simulink model "final_quadruped_120722"  (R2021a)
settings: Solver=ode15s  StartTime=0.0  StopTime=10  FixedStep=1e-3  RelTol=1e-5  EnableMultiTasking=on
values from neighbouring files (symbols this model uses):
  foot_x = 8    [bipedparameters.m]    (also in fcn.m; finalrobotParameters.m; finalrobotParameters_110522.m; finalrobotParameters_140522.m)
  foot_y = 6    [bipedparameters.m]    (also in fcn.m; finalrobotParameters.m; finalrobotParameters_110522.m; finalrobotParameters_140522.m)
  foot_z = 1    [bipedparameters.m]    (also in fcn.m; finalrobotParameters.m; finalrobotParameters_110522.m; finalrobotParameters_140522.m)
  height_plane = 0.025    [bipedparameters.m]    (also in finalrobotParameters.m; finalrobotParameters_110522.m; finalrobotParameters_140522.m; finalrobotParameters_240522.m)
  kd_ankle = 1000    [bipedparameters.m]    (also in finalrobotParameters_240522.m)
  kd_hip = 1000    [bipedparameters.m]    (also in finalrobotParameters_240522.m)
  kd_knee = 1000    [bipedparameters.m]    (also in finalrobotParameters_240522.m)
  ki_ankle = 1000    [bipedparameters.m]    (also in finalrobotParameters_240522.m)
  ki_hip = 1000    [bipedparameters.m]    (also in finalrobotParameters_240522.m)
  ki_knee = 2000    [bipedparameters.m]    (also in finalrobotParameters_240522.m)
  kp_ankle = 1000    [bipedparameters.m]    (also in finalrobotParameters_240522.m)
  kp_hip = 1000    [bipedparameters.m]    (also in finalrobotParameters_240522.m)
  kp_knee = 2000    [bipedparameters.m]    (also in finalrobotParameters_240522.m)
  lower_leg_length = 10    [bipedparameters.m]    (also in fcn.m; finalrobotParameters.m; finalrobotParameters_110522.m; finalrobotParameters_140522.m)
  plane_x = 25    [bipedparameters.m]    (also in finalrobotParameters.m; finalrobotParameters_110522.m; finalrobotParameters_140522.m; finalrobotParameters_240522.m)
  plane_y = 3    [bipedparameters.m]    (also in finalrobotParameters.m; finalrobotParameters_110522.m; finalrobotParameters_140522.m; finalrobotParameters_240522.m)
  torso_offset_x = -0.5    [bipedparameters.m]    (also in finalrobotParameters.m = 10; finalrobotParameters_110522.m = 10; finalrobotParameters_140522.m = 10; finalrobotParameters_240522.m = 10)
  torso_offset_z = -2    [bipedparameters.m]    (also in finalrobotParameters.m; finalrobotParameters_110522.m; finalrobotParameters_140522.m; finalrobotParameters_240522.m)
  torso_x = 5    [bipedparameters.m]    (also in fcn.m = 25; finalrobotParameters.m = 25; finalrobotParameters_110522.m = 25; finalrobotParameters_140522.m = 25)
  torso_y = 10    [bipedparameters.m]    (also in fcn.m = 16; finalrobotParameters.m = 16; finalrobotParameters_110522.m = 16; finalrobotParameters_140522.m = 16)
  torso_z = 8    [bipedparameters.m]    (also in fcn.m = 10; finalrobotParameters.m = 10; finalrobotParameters_110522.m = 10; finalrobotParameters_140522.m = 10)
  upper_leg_length = 10    [bipedparameters.m]    (also in fcn.m; finalrobotParameters.m; finalrobotParameters_110522.m; finalrobotParameters_140522.m)
undefined symbols (not defined in the file or in its folder): sigbuilder_block, X, Y, Z
libraries: nesl_utility x288, sm_lib x75, pid_lib x20, Contact_Forces_Lib x16, fl_lib x3
(part 4 of 9)

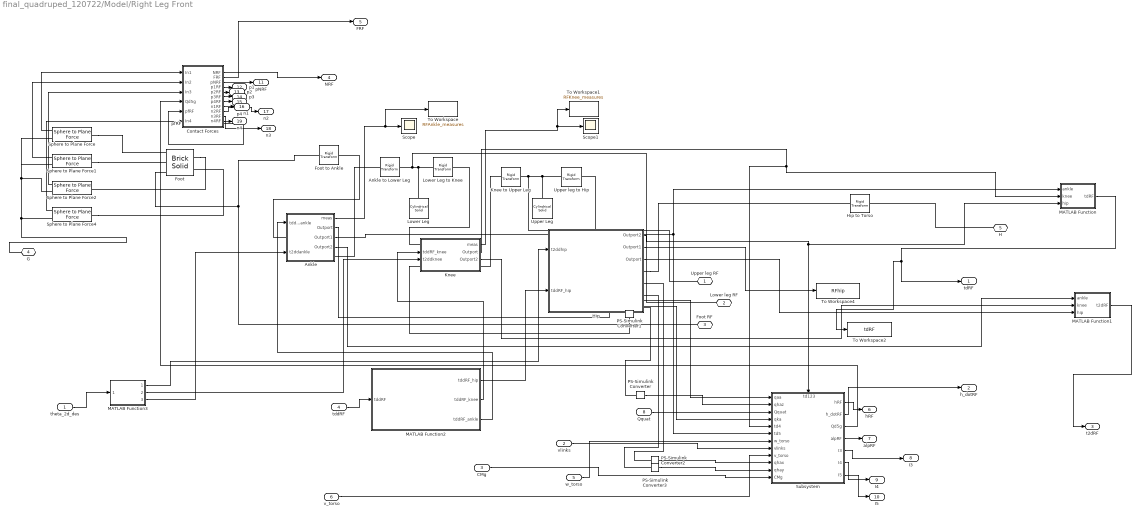
== system final_quadruped_120722/Model/Right Leg Front  ==
  theta_2d_des : Inport
  vlinks : Inport  Port=2
  CMg : Inport  Port=3
  tddRF : Inport  Port=4
  w_torso : Inport  Port=5
  v_torso : Inport  Port=6
  pfRF : Inport  Port=7
  Qquat : Inport  Port=8
  "Ankle " : Subsystem
      settings: PortSchema="{\"entries\":[{\"content\":{\"sides\":[{\"content\":{\"connectorIds\":[\"In1\",\"LConn1\",\"In2\"]},\"type\":\"ConnectorPlacement.EquallySpacedRectSide\",\"uuid\":\"8820d672-3cef-4e81-999d-8ce69d7112c4\"},{\"content\":{\"connectorIds\":[\"Out1\",\"Out2\",\"Out3\",\"Out4\",\"RConn1\"],\"side\":\"RIGHT\"},\"type\":\"ConnectorPlacement.EquallySpacedRectSide\",\"uuid\":\"2ab010ff-dc37-45a7-8249-0a0b10f28039\"},{\"content\":{\"connectorIds\":[],\"side\":\"TOP\"},\"type\":\"ConnectorPlacement.EquallySpacedRectSide\",\"uuid\":\"2949f9ef-a473-4fca-9f6b-f5ba56dbec95\"}]},\"type\":\"ConnectorPlacement.EquallySpacedConnector\",\"uuid\":\"7b6aa300-a222-434d-a157-d54fa47a17c2\"}],\"packageUris\":[\"http://schema.mathworks.com/mf0/Connector/R2020b\"],\"version\":\"1.0\"}"
  Ankle to Lower Leg : sm_lib/Frames and Transforms/Rigid Transform  TranslationMethod=Cartesian  TranslationStandardOffset=5  TranslationLengthUnit=cm  TranslationStandardAxis=+Y  TranslationCartesianOffset=[0 lower_leg_length/2 0]  TranslationROffset=0  TranslationROffsetUnits=m  TranslationZOffset=0  TranslationZOffsetUnits=m  TranslationThetaOffset=0  TranslationThetaOffsetUnits=deg  RotationMethod=StandardAxis  RotationAngleUnits=deg  RotationStandardAxis=-X  RotationAngle=90  RotationArbitraryAxis=[0 0 1]  FollAlignAxisA=+X  BaseAlignAxisA=+Y  FollAlignAxisB=+Y  BaseAlignAxisB=+Z  RotationSequenceAxes=FollowerAxes  RotationSequence=XYX  RotationSequenceAngles=[0 0 0]  RotationSequenceAnglesUnits=deg  RotationMatrix=[1 0 0; 0 1 0; 0 0 1]
  "Contact Forces " : Subsystem
  Foot : sm_lib/Body Elements/Brick Solid  GraphicAmbientColor=[0.15 0.15 0.15 1.0]  BasedOnType=Density  BrickDimensions=[foot_x foot_y foot_z]  BrickDimensionUnits=cm  CenterOfMass=[0 0 0]  CenterOfMassUnits=m  GraphicDiffuseColor=[0.5 0.5 0.5]  Density=foot_density  DensityUnits=kg/m^3  DoExposeReferenceFrame=off  GraphicEmissiveColor=[0.0 0.0 0.0 1.0]  ExportEntireGeometry=off  SerializedFrames=<Frames><Frame><Id>Frame1</Id><Value><Name>F1</Name><Origin><Source>GeometricFeature</Source><FeatureName>+x -y -z point</FeatureName></Origin><PrimaryAxis><DefinedDirection>+Z</DefinedDirection><Source>ReferenceFrame</Source><SourceDirection>+Z</SourceDirection><FeatureName></FeatureName></PrimaryAxis><SecondaryAxis><DefinedDirection>+X</DefinedDirection><Source>ReferenceFrame</Source><SourceDirection>+X</SourceDirection><FeatureName></FeatureName></SecondaryAxis></Value></Frame><Frame><Id>Frame2</Id><Value><Name>F2</Name><Origin><Source>GeometricFeature</Source><FeatureName>-x -y -z point</FeatureName></Origin><PrimaryAxis><DefinedDirection>+Z</DefinedDirection><Source>ReferenceFrame</Source><SourceDirection>+Z</SourceDirection><FeatureName></FeatureName></PrimaryAxis><SecondaryAxis><DefinedDirection>+X</DefinedDirection><Source>ReferenceFrame</Source><SourceDirection>+X</SourceDirection><FeatureName></FeatureName></SecondaryAxis></Value></Frame><Frame><Id>Frame3</Id><Value><Name>F3</Name><Origin><Source>GeometricFeature</Source><FeatureName>+x +y -z point</FeatureName></Origin><PrimaryAxis><DefinedDirection>+Z</DefinedDirection><Source>ReferenceFrame</Source><SourceDirection>+Z</SourceDirection><FeatureName></FeatureName></PrimaryAxis><SecondaryAxis><DefinedDirection>+X</DefinedDirection><Source>ReferenceFrame</Source><SourceDirection>+X</SourceDirection><FeatureName></FeatureName></SecondaryAxis></Value></Frame><Frame><Id>Frame4</Id><Value><Name>F4</Name><Origin><Source>GeometricFeature</Source><FeatureName>-x +y -z point</FeatureName></Origin><PrimaryAxis><DefinedDirection>+Z</DefinedDirection><Source>ReferenceFrame</Source><SourceDirection>+Z</SourceDirection><FeatureName></FeatureName></PrimaryAxis><SecondaryAxis><DefinedDirection>+X</DefinedDirection><Source>ReferenceFrame</Source><SourceDirection>+X</SourceDirection><FeatureName></FeatureName></SecondaryAxis></Value></Frame><Frame><Id>Frame5</Id><Value><Name>B</Name><Origin><Source>GeometricFeature</Source><FeatureName>+z surface</FeatureName></Origin><PrimaryAxis><DefinedDirection>+Z</DefinedDirection><Source>ReferenceFrame</Source><SourceDirection>-Y</SourceDirection><FeatureName></FeatureName></PrimaryAxis><SecondaryAxis><DefinedDirection>+X</DefinedDirection><Source>ReferenceFrame</Source><SourceDirection>+X</SourceDirection><FeatureName></FeatureName></SecondaryAxis></Value></Frame></Frames>  MarkerShape=Sphere  MarkerSize=10  GraphicType=FromGeometry  InertiaType=CalculateFromGeometry  Mass=1  MassUnits=kg  MomentsOfInertia=[1 1 1]  MomentsOfInertiaUnits=kg*m^2  GraphicOpacity=1.0  ProductsOfInertia=[1 1 1]  ProductsOfInertiaUnits=kg*m^2  GraphicShininess=75  GraphicSpecularColor=[0.5 0.5 0.5 1.0]  GraphicVisPropType=SimpleVisualProperties
  Foot to Ankle : sm_lib/Frames and Transforms/Rigid Transform  TranslationMethod=Cartesian  TranslationStandardOffset=0  TranslationLengthUnit=cm  TranslationStandardAxis=+Z  TranslationCartesianOffset=foot_offset  TranslationROffset=0  TranslationROffsetUnits=m  TranslationZOffset=0  TranslationZOffsetUnits=m  TranslationThetaOffset=0  TranslationThetaOffsetUnits=deg  RotationMethod=None  RotationAngleUnits=deg  RotationStandardAxis=+X  RotationAngle=90  RotationArbitraryAxis=[0 0 1]  FollAlignAxisA=+X  BaseAlignAxisA=+Y  FollAlignAxisB=+Y  BaseAlignAxisB=+Z  RotationSequenceAxes=FollowerAxes  RotationSequence=XYX  RotationSequenceAngles=[0 0 0]  RotationSequenceAnglesUnits=deg  RotationMatrix=[1 0 0; 0 1 0; 0 0 1]
  Hip : Subsystem
      settings: PortSchema="{\"entries\":[{\"content\":{\"sides\":[{\"content\":{\"connectorIds\":[\"In1\",\"In2\"]},\"type\":\"ConnectorPlacement.EquallySpacedRectSide\",\"uuid\":\"3c672348-e331-4589-83a8-aa84cb04ec22\"},{\"content\":{\"connectorIds\":[\"Out1\",\"Out2\",\"Out3\",\"RConn1\",\"RConn2\",\"RConn3\",\"RConn4\"],\"side\":\"RIGHT\"},\"type\":\"ConnectorPlacement.EquallySpacedRectSide\",\"uuid\":\"0cc20eac-f861-4ef7-921b-23889a7eea47\"},{\"content\":{\"connectorIds\":[\"LConn1\"],\"side\":\"TOP\"},\"type\":\"ConnectorPlacement.EquallySpacedRectSide\",\"uuid\":\"90940c46-a35e-4cbd-8c5c-08301adb8b47\"}]},\"type\":\"ConnectorPlacement.EquallySpacedConnector\",\"uuid\":\"ac1266b5-f3f5-41bb-99c9-3c0745f7848a\"}],\"packageUris\":[\"http://schema.mathworks.com/mf0/Connector/R2020b\"],\"version\":\"1.0\"}"
  Hip to Torso : sm_lib/Frames and Transforms/Rigid Transform  TranslationMethod=None  TranslationStandardOffset=0  TranslationLengthUnit=m  TranslationStandardAxis=+Z  TranslationCartesianOffset=[0 0 0]  TranslationROffset=0  TranslationROffsetUnits=m  TranslationZOffset=0  TranslationZOffsetUnits=m  TranslationThetaOffset=0  TranslationThetaOffsetUnits=deg  RotationMethod=StandardAxis  RotationAngleUnits=deg  RotationStandardAxis=+X  RotationAngle=-90  RotationArbitraryAxis=[0 0 1]  FollAlignAxisA=+X  BaseAlignAxisA=+Y  FollAlignAxisB=+Y  BaseAlignAxisB=+Z  RotationSequenceAxes=FollowerAxes  RotationSequence=XYX  RotationSequenceAngles=[0 0 0]  RotationSequenceAnglesUnits=deg  RotationMatrix=[1 0 0; 0 1 0; 0 0 1]
  Knee : Subsystem
      settings: PortSchema="{\"entries\":[{\"content\":{\"sides\":[{\"content\":{\"connectorIds\":[\"LConn1\",\"In1\",\"In2\",\"LConn2\"]},\"type\":\"ConnectorPlacement.EquallySpacedRectSide\",\"uuid\":\"3c672348-e331-4589-83a8-aa84cb04ec22\"},{\"content\":{\"connectorIds\":[\"Out1\",\"Out2\",\"Out3\",\"RConn1\"],\"side\":\"RIGHT\"},\"type\":\"ConnectorPlacement.EquallySpacedRectSide\",\"uuid\":\"0cc20eac-f861-4ef7-921b-23889a7eea47\"},{\"content\":{\"connectorIds\":[],\"side\":\"TOP\"},\"type\":\"ConnectorPlacement.EquallySpacedRectSide\",\"uuid\":\"90940c46-a35e-4cbd-8c5c-08301adb8b47\"}]},\"type\":\"ConnectorPlacement.EquallySpacedConnector\",\"uuid\":\"ac1266b5-f3f5-41bb-99c9-3c0745f7848a\"}],\"packageUris\":[\"http://schema.mathworks.com/mf0/Connector/R2020b\"],\"version\":\"1.0\"}"
  Knee to Upper Leg : sm_lib/Frames and Transforms/Rigid Transform  TranslationMethod=Cartesian  TranslationStandardOffset=5  TranslationLengthUnit=cm  TranslationStandardAxis=+Y  TranslationCartesianOffset=[0 upper_leg_length/2 0]  TranslationROffset=0  TranslationROffsetUnits=m  TranslationZOffset=0  TranslationZOffsetUnits=m  TranslationThetaOffset=0  TranslationThetaOffsetUnits=deg  RotationMethod=StandardAxis  RotationAngleUnits=deg  RotationStandardAxis=+X  RotationAngle=-90  RotationArbitraryAxis=[0 0 1]  FollAlignAxisA=+X  BaseAlignAxisA=+Y  FollAlignAxisB=+Y  BaseAlignAxisB=+Z  RotationSequenceAxes=FollowerAxes  RotationSequence=XYX  RotationSequenceAngles=[0 0 0]  RotationSequenceAnglesUnits=deg  RotationMatrix=[1 0 0; 0 1 0; 0 0 1]
  Lower Leg : sm_lib/Body Elements/Cylindrical Solid  GraphicAmbientColor=[0.15 0.15 0.15 1.0]  BasedOnType=Density  CenterOfMass=[0 0 0]  CenterOfMassUnits=m  GraphicDiffuseColor=[0.5 0.5 0.5]  CylinderLength=lower_leg_length  CylinderLengthUnits=cm  CylinderRadius=leg_radius  CylinderRadiusUnits=cm  Density=density  DensityUnits=kg/m^3  DoExposeReferenceFrame=on  GraphicEmissiveColor=[0.0 0.0 0.0 1.0]  ExportEntireGeometry=off  SerializedFrames=<Frames/>  MarkerShape=Sphere  MarkerSize=10  GraphicType=FromGeometry  InertiaType=CalculateFromGeometry  Mass=1  MassUnits=kg  MomentsOfInertia=[1 1 1]  MomentsOfInertiaUnits=kg*m^2  GraphicOpacity=1.0  ProductsOfInertia=[1 1 1]  ProductsOfInertiaUnits=kg*m^2  GraphicShininess=75  GraphicSpecularColor=[0.5 0.5 0.5 1.0]  GraphicVisPropType=SimpleVisualProperties
  Lower Leg to Knee : sm_lib/Frames and Transforms/Rigid Transform  TranslationMethod=Cartesian  TranslationStandardOffset=5  TranslationLengthUnit=cm  TranslationStandardAxis=+Z  TranslationCartesianOffset=[0 0 lower_leg_length/2]  TranslationROffset=0  TranslationROffsetUnits=m  TranslationZOffset=0  TranslationZOffsetUnits=m  TranslationThetaOffset=0  TranslationThetaOffsetUnits=deg  RotationMethod=StandardAxis  RotationAngleUnits=deg  RotationStandardAxis=+X  RotationAngle=90  RotationArbitraryAxis=[0 0 1]  FollAlignAxisA=+X  BaseAlignAxisA=+Y  FollAlignAxisB=+Y  BaseAlignAxisB=+Z  RotationSequenceAxes=FollowerAxes  RotationSequence=XYX  RotationSequenceAngles=[0 0 0]  RotationSequenceAnglesUnits=deg  RotationMatrix=[1 0 0; 0 1 0; 0 0 1]
  MATLAB Function : MATLAB Function  TreatAsAtomicUnit=on
  MATLAB Function1 : MATLAB Function  TreatAsAtomicUnit=on
  MATLAB Function2 : MATLAB Function  TreatAsAtomicUnit=on
  MATLAB Function3 : MATLAB Function  TreatAsAtomicUnit=on
  PS-Simulink Converter{,1..3} (4 alike) : nesl_utility/PS-Simulink Converter  PhysicalDomain=network_engine_domain  SubClassName=ps_output  LeftPortType=input  RightPortType=output  PseudoPeriodic=off  Frequencies=[]  Unit=inherit  AffineConversion=off
      settings: SourceProductBaseCode=PW,SS
  Scope : Scope
  Scope1 : Scope
  Sphere to Plane Force : Contact_Forces_Lib/3D/Sphere to Plane Force  sphere_rad=contact_point_radius  plane_lenx=plane_x  plane_leny=plane_y  plane_depth=height_plane/2  force_law=Linear  k_contact=contact_stiffness  b_contact=contact_damping  pen_full_damp_F=1e-4  pen_exponent=1  custom_param_1=1  custom_param_2=1  friction_law=Stick-Slip Continuous  mu_kinetic=mu_k  mu_static=mu_s  v_thr=mu_vth  vis_on=on  vis_opc_en=0  vis_len_plaBz=0.005  vis_clr=[0.9 0.2 0.2]  vis_opc=0.7
  Sphere to Plane Force1 : Contact_Forces_Lib/3D/Sphere to Plane Force  sphere_rad=contact_point_radius  plane_lenx=plane_x  plane_leny=plane_y  plane_depth=height_plane/2  force_law=Linear  k_contact=contact_stiffness  b_contact=contact_damping  pen_full_damp_F=1e-4  pen_exponent=1  custom_param_1=1  custom_param_2=1  friction_law=Stick-Slip Continuous  mu_kinetic=mu_k  mu_static=mu_s  v_thr=mu_vth  vis_on=off  vis_opc_en=0  vis_len_plaBz=0.005  vis_clr=[0.9 0.2 0.2]  vis_opc=0.7
  Sphere to Plane Force2 : Contact_Forces_Lib/3D/Sphere to Plane Force  sphere_rad=contact_point_radius  plane_lenx=plane_x  plane_leny=plane_y  plane_depth=height_plane/2  force_law=Linear  k_contact=contact_stiffness  b_contact=contact_damping  pen_full_damp_F=1e-4  pen_exponent=1  custom_param_1=1  custom_param_2=1  friction_law=Stick-Slip Continuous  mu_kinetic=mu_k  mu_static=mu_s  v_thr=mu_vth  vis_on=off  vis_opc_en=0  vis_len_plaBz=0.005  vis_clr=[0.9 0.2 0.2]  vis_opc=0.7
  Sphere to Plane Force4 : Contact_Forces_Lib/3D/Sphere to Plane Force  sphere_rad=contact_point_radius  plane_lenx=plane_x  plane_leny=plane_y  plane_depth=height_plane/2  force_law=Linear  k_contact=contact_stiffness  b_contact=contact_damping  pen_full_damp_F=1e-4  pen_exponent=1  custom_param_1=1  custom_param_2=1  friction_law=Stick-Slip Continuous  mu_kinetic=mu_k  mu_static=mu_s  v_thr=mu_vth  vis_on=off  vis_opc_en=0  vis_len_plaBz=0.005  vis_clr=[0.9 0.2 0.2]  vis_opc=0.7
  Subsystem : Subsystem
      settings: PortSchema="{\"entries\":[{\"content\":{\"sides\":[{\"content\":{\"connectorIds\":[\"In1\",\"In2\",\"In3\",\"In4\",\"In5\",\"In6\",\"In7\",\"In8\",\"In9\",\"In10\",\"In11\",\"In12\"]},\"type\":\"ConnectorPlacement.EquallySpacedRectSide\",\"uuid\":\"86ce1042-93a3-4257-9482-b934ed56108e\"},{\"content\":{\"connectorIds\":[\"Out1\",\"Out2\",\"Out3\",\"Out4\",\"Out5\",\"Out6\",\"Out7\"],\"side\":\"RIGHT\"},\"type\":\"ConnectorPlacement.EquallySpacedRectSide\",\"uuid\":\"9186dd22-c036-4814-9c8f-a02c82466cca\"},{\"content\":{\"connectorIds\":[\"In13\"],\"side\":\"TOP\"},\"type\":\"ConnectorPlacement.EquallySpacedRectSide\",\"uuid\":\"8b91f2be-4c09-4acb-8fc1-b217aa758295\"}]},\"type\":\"ConnectorPlacement.EquallySpacedConnector\",\"uuid\":\"b7c3f053-f66c-40d9-bf5a-575a18fb37e5\"}],\"packageUris\":[\"http://schema.mathworks.com/mf0/Connector/R2020b\"],\"version\":\"1.0\"}"
  To Workspace : ToWorkspace  VariableName=RFAnkle_measures  SaveFormat=Timeseries  SampleTime=-1
  To Workspace1 : ToWorkspace  VariableName=RFKnee_measures  SaveFormat=Timeseries  SampleTime=-1
  To Workspace2 : ToWorkspace  VariableName=tdRF  SaveFormat=Timeseries  SampleTime=-1
  To Workspace4 : ToWorkspace  VariableName=RFhip  SaveFormat=Timeseries  SampleTime=-1
  Upper Leg : sm_lib/Body Elements/Cylindrical Solid  GraphicAmbientColor=[0.15 0.15 0.15 1.0]  BasedOnType=Density  CenterOfMass=[0 0 0]  CenterOfMassUnits=m  GraphicDiffuseColor=[0.5 0.5 0.5]  CylinderLength=upper_leg_length  CylinderLengthUnits=cm  CylinderRadius=leg_radius  CylinderRadiusUnits=cm  Density=1000  DensityUnits=kg/m^3  DoExposeReferenceFrame=on  GraphicEmissiveColor=[0.0 0.0 0.0 1.0]  ExportEntireGeometry=off  SerializedFrames=<Frames/>  MarkerShape=Sphere  MarkerSize=10  GraphicType=FromGeometry  InertiaType=CalculateFromGeometry  Mass=1  MassUnits=kg  MomentsOfInertia=[1 1 1]  MomentsOfInertiaUnits=kg*m^2  GraphicOpacity=1.0  ProductsOfInertia=[1 1 1]  ProductsOfInertiaUnits=kg*m^2  GraphicShininess=75  GraphicSpecularColor=[0.5 0.5 0.5 1.0]  GraphicVisPropType=SimpleVisualProperties
  Upper leg to Hip : sm_lib/Frames and Transforms/Rigid Transform  TranslationMethod=Cartesian  TranslationStandardOffset=5  TranslationLengthUnit=cm  TranslationStandardAxis=+Z  TranslationCartesianOffset=[0 0 upper_leg_length/2]  TranslationROffset=0  TranslationROffsetUnits=m  TranslationZOffset=0  TranslationZOffsetUnits=m  TranslationThetaOffset=0  TranslationThetaOffsetUnits=deg  RotationMethod=StandardAxis  RotationAngleUnits=deg  RotationStandardAxis=+X  RotationAngle=90  RotationArbitraryAxis=[0 0 1]  FollAlignAxisA=+X  BaseAlignAxisA=+Y  FollAlignAxisB=+Y  BaseAlignAxisB=+Z  RotationSequenceAxes=FollowerAxes  RotationSequence=XYX  RotationSequenceAngles=[0 0 0]  RotationSequenceAnglesUnits=deg  RotationMatrix=[1 0 0; 0 1 0; 0 0 1]
  Upper leg RF : PMIOPort  Side=Left
  Lower leg RF : PMIOPort  Port=2  Side=Left
  Foot RF : PMIOPort  Port=3  Side=Left
  "G " : PMIOPort  Port=4  Side=Right
  H : PMIOPort  Port=5  Side=Right
  tdRF : Outport
  h_dotRF : Outport  Port=2
  t2dRF : Outport  Port=3
  NRF : Outport  Port=4
  FRF : Outport  Port=5
  hRF : Outport  Port=6
  alpRF : Outport  Port=7
  I3 : Outport  Port=8
  I4 : Outport  Port=9
  I5 : Outport  Port=10
  pNRF : Outport  Port=11
  p1 : Outport  Port=12
  p2 : Outport  Port=13
  p3 : Outport  Port=14
  p4 : Outport  Port=15
  n1 : Outport  Port=16
  n2 : Outport  Port=17
  n3 : Outport  Port=18
  n4 : Outport  Port=19
  wires:
  Sphere to Plane Force/1 -> "Contact Forces "/1(In1)
  Sphere to Plane Force1/1 -> "Contact Forces "/2(In2)
  Sphere to Plane Force2/1 -> "Contact Forces "/3(In3)
  Sphere to Plane Force4/1 -> "Contact Forces "/6(In4)
  "Ankle "/1(meas) -> To Workspace/1, Scope/1
  tddRF/1 -> MATLAB Function2/1(tddRF)
  MATLAB Function2/3(tddRF_ankle) -> "Ankle "/1(tddRF_ankle)
  Knee/1(meas) -> To Workspace1/1, Scope1/1
  MATLAB Function2/2(tddRF_knee) -> Knee/1(tddRF_knee)
  MATLAB Function2/1(tddRF_hip) -> Hip/2(tddRF_hip)
  "Ankle "/2(Outport) -> Subsystem/1(qaa)
  Qquat/1 -> Subsystem/3(Qquat)
  PS-Simulink Converter1/1 -> Subsystem/4(qka)
  "Ankle "/3(Outport1) -> Subsystem/6(td5), MATLAB Function/1(ankle)
  Knee/2(Outport) -> MATLAB Function/2(knee), Subsystem/5(td4)
  MATLAB Function/1(tdRF) -> To Workspace2/1, tdRF/1
  w_torso/1 -> Subsystem/7(w_torso)
  v_torso/1 -> Subsystem/9(v_torso)
  vlinks/1 -> Subsystem/8(vlinks)
  Subsystem/2(h_dotRF) -> h_dotRF/1
  "Ankle "/4(Outport2) -> MATLAB Function1/1(ankle)
  Knee/3(Outport2) -> MATLAB Function1/2(knee)
  Hip/1(Outport2) -> Subsystem/13(td123), MATLAB Function/3(hip)
  MATLAB Function1/1(t2dRF) -> t2dRF/1
  "Contact Forces "/1(NRF) -> NRF/1
  "Contact Forces "/2(FRF) -> FRF/1
  theta_2d_des/1 -> MATLAB Function3/1(theta_2d_des)
  MATLAB Function3/3(t2ddankle) -> "Ankle "/2(t2ddankle)
  MATLAB Function3/2(t2ddknee) -> Knee/2(t2ddknee)
  MATLAB Function3/1(t2ddhip) -> Hip/1(t2ddhip)
  Subsystem/3(Qd5g) -> "Contact Forces "/4(Qd5g)
  PS-Simulink Converter2/1 -> Subsystem/10(qhax)
  PS-Simulink Converter3/1 -> Subsystem/11(qhay)
  PS-Simulink Converter/1 -> Subsystem/2(qhaz)
  Hip/2(Outport1) -> To Workspace4/1
  Hip/3(Outport) -> MATLAB Function1/3(hip)
  CMg/1 -> Subsystem/12(CMg)
  Subsystem/1(hRF) -> hRF/1
  Subsystem/4(alpRF) -> alpRF/1
  Subsystem/5(I3) -> I3/1
  Subsystem/6(I4) -> I4/1
  Subsystem/7(I5) -> I5/1
  pfRF/1 -> "Contact Forces "/5(pfRF)
  "Contact Forces "/3(pNRF) -> pNRF/1
  "Contact Forces "/4(p1RF) -> p1/1
  "Contact Forces "/5(p2RF) -> p2/1
  "Contact Forces "/6(p3RF) -> p3/1
  "Contact Forces "/7(p4RF) -> p4/1
  "Contact Forces "/8(n1RF) -> n1/1
  "Contact Forces "/9(n2RF) -> n2/1
  "Contact Forces "/10(n3RF) -> n3/1
  "Contact Forces "/11(n4RF) -> n4/1
  connections:
  H/RConn1 -- Hip to Torso/RConn1
  Lower Leg to Knee/LConn1 -- Lower Leg/RConn1 -- Lower leg RF/RConn1 -- Ankle to Lower Leg/RConn1
  Upper leg to Hip/LConn1 -- Upper Leg/RConn1 -- Upper leg RF/RConn1 -- Knee to Upper Leg/RConn1
  Sphere to Plane Force/LConn1 -- Foot/LConn1
  Sphere to Plane Force1/LConn1 -- Foot/LConn2
  Sphere to Plane Force4/LConn1 -- Foot/RConn2
  Sphere to Plane Force2/RConn1 -- Sphere to Plane Force1/RConn1 -- Sphere to Plane Force/RConn1 -- Sphere to Plane Force4/RConn1 -- "G "/RConn1
  "Ankle "/LConn1 -- Foot to Ankle/RConn1
  Ankle to Lower Leg/LConn1 -- "Ankle "/RConn1
  Foot/RConn1 -- Sphere to Plane Force2/LConn1
  Foot/LConn3 -- Foot to Ankle/LConn1 -- Foot RF/RConn1
  Knee/LConn1 -- Lower Leg to Knee/RConn1
  Knee to Upper Leg/LConn1 -- Knee/RConn1
  PS-Simulink Converter1/LConn1 -- Knee/LConn2
  Hip/LConn1 -- Upper leg to Hip/RConn1
  Hip/RConn1 -- Hip to Torso/LConn1
  PS-Simulink Converter2/LConn1 -- Hip/RConn2
  PS-Simulink Converter3/LConn1 -- Hip/RConn3
  PS-Simulink Converter/LConn1 -- Hip/RConn4

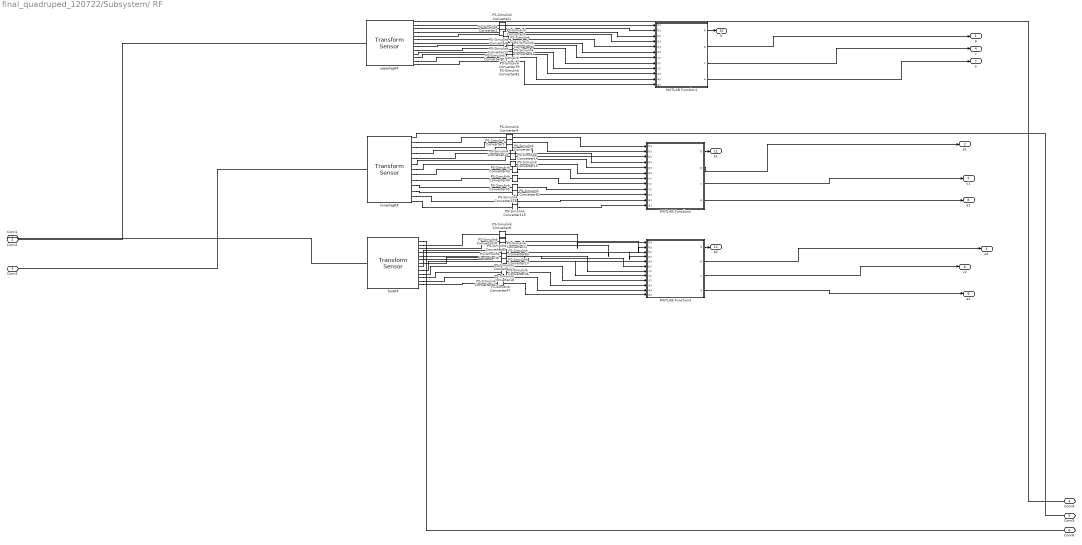
== system final_quadruped_120722/Subsystem/ RF ==
  MATLAB Function1 : MATLAB Function  TreatAsAtomicUnit=on
  MATLAB Function2 : MATLAB Function  TreatAsAtomicUnit=on
  MATLAB Function3 : MATLAB Function  TreatAsAtomicUnit=on
  PS-Simulink Converter{1..18,40..48,79..85,115..116} (36 alike) : nesl_utility/PS-Simulink Converter  PhysicalDomain=network_engine_domain  SubClassName=ps_output  LeftPortType=input  RightPortType=output  PseudoPeriodic=off  Frequencies=[]  Unit=inherit  AffineConversion=off
      settings: SourceProductBaseCode=PW,SS
  footRF : sm_lib/Frames and Transforms/Transform Sensor  MeasurementFrame=World  SenseAngle=off  SenseAxis=off  SenseAngle1=off  SenseAngle2=off  SenseAngle3=off  SenseQ=off  SenseR=off  SenseOmegaX=off  SenseOmegaY=off  SenseOmegaZ=off  SenseOmega1=off  SenseOmega2=off  SenseOmega3=off  SenseQDot=off  SenseRDot=off  SenseAlphaX=on  SenseAlphaY=on  SenseAlphaZ=on  SenseAlpha1=off  SenseAlpha2=off  SenseAlpha3=off  SenseQDDot=off  SenseRDDot=off  SenseX=on  SenseY=on  SenseZ=on  SenseRad=off  SenseAzim=off  SenseDist=off  SenseInc=off  SenseXDot=on  SenseYDot=on  SenseZDot=on  SenseRadDot=off  SenseAzimDot=off  SenseDistDot=off  SenseIncDot=off  SenseXDDot=on  SenseYDDot=on  SenseZDDot=on  SenseRadDDot=off  SenseAzimDDot=off  SenseDistDDot=off  SenseIncDDot=off
  lowerlegRF : sm_lib/Frames and Transforms/Transform Sensor  MeasurementFrame=World  SenseAngle=off  SenseAxis=off  SenseAngle1=off  SenseAngle2=off  SenseAngle3=off  SenseQ=off  SenseR=off  SenseOmegaX=off  SenseOmegaY=off  SenseOmegaZ=off  SenseOmega1=off  SenseOmega2=off  SenseOmega3=off  SenseQDot=off  SenseRDot=off  SenseAlphaX=on  SenseAlphaY=on  SenseAlphaZ=on  SenseAlpha1=off  SenseAlpha2=off  SenseAlpha3=off  SenseQDDot=off  SenseRDDot=off  SenseX=on  SenseY=on  SenseZ=on  SenseRad=off  SenseAzim=off  SenseDist=off  SenseInc=off  SenseXDot=on  SenseYDot=on  SenseZDot=on  SenseRadDot=off  SenseAzimDot=off  SenseDistDot=off  SenseIncDot=off  SenseXDDot=on  SenseYDDot=on  SenseZDDot=on  SenseRadDDot=off  SenseAzimDDot=off  SenseDistDDot=off  SenseIncDDot=off
  upperlegRF : sm_lib/Frames and Transforms/Transform Sensor  MeasurementFrame=World  SenseAngle=off  SenseAxis=off  SenseAngle1=off  SenseAngle2=off  SenseAngle3=off  SenseQ=off  SenseR=off  SenseOmegaX=off  SenseOmegaY=off  SenseOmegaZ=off  SenseOmega1=off  SenseOmega2=off  SenseOmega3=off  SenseQDot=off  SenseRDot=off  SenseAlphaX=on  SenseAlphaY=on  SenseAlphaZ=on  SenseAlpha1=off  SenseAlpha2=off  SenseAlpha3=off  SenseQDDot=off  SenseRDDot=off  SenseX=on  SenseY=on  SenseZ=on  SenseRad=off  SenseAzim=off  SenseDist=off  SenseInc=off  SenseXDot=on  SenseYDot=on  SenseZDot=on  SenseRadDot=off  SenseAzimDot=off  SenseDistDot=off  SenseIncDot=off  SenseXDDot=on  SenseYDDot=on  SenseZDDot=on  SenseRadDDot=off  SenseAzimDDot=off  SenseDistDDot=off  SenseIncDDot=off
  Conn1 : PMIOPort  Side=Left
  Conn2 : PMIOPort  Port=2  Side=Left
  Conn3 : PMIOPort  Port=3  Side=Left
  Conn4 : PMIOPort  Port=4  Side=Right
  Conn5 : PMIOPort  Port=5  Side=Right
  Conn6 : PMIOPort  Port=6  Side=Right
  p : Outport
  p1 : Outport  Port=2
  p2 : Outport  Port=3
  v : Outport  Port=4
  v1 : Outport  Port=5
  v2 : Outport  Port=6
  a : Outport  Port=7
  a1 : Outport  Port=8
  a2 : Outport  Port=9
  b : Outport  Port=10
  b1 : Outport  Port=11
  b2 : Outport  Port=12
  wires:
  PS-Simulink Converter116/1 -> MATLAB Function2/12(az)
  PS-Simulink Converter17/1 -> MATLAB Function3/8(vy)
  MATLAB Function2/4(a) -> a1/1
  PS-Simulink Converter79/1 -> MATLAB Function1/10(ax)
  PS-Simulink Converter16/1 -> MATLAB Function3/7(vx)
  PS-Simulink Converter6/1 -> MATLAB Function1/4(px)
  PS-Simulink Converter84/1 -> MATLAB Function3/5(py)
  PS-Simulink Converter13/1 -> MATLAB Function2/4(px)
  PS-Simulink Converter82/1 -> MATLAB Function2/10(ax)
  PS-Simulink Converter47/1 -> MATLAB Function3/11(ay)
  PS-Simulink Converter18/1 -> MATLAB Function3/9(vz)
  PS-Simulink Converter83/1 -> MATLAB Function3/4(px)
  PS-Simulink Converter15/1 -> MATLAB Function2/6(pz)
  PS-Simulink Converter42/1 -> MATLAB Function1/9(vz)
  PS-Simulink Converter45/1 -> MATLAB Function2/9(vz)
  MATLAB Function3/4(a) -> a2/1
  MATLAB Function1/2(p) -> p/1
  PS-Simulink Converter43/1 -> MATLAB Function2/7(vx)
  PS-Simulink Converter85/1 -> MATLAB Function3/6(pz)
  PS-Simulink Converter44/1 -> MATLAB Function2/8(vy)
  PS-Simulink Converter12/1 -> MATLAB Function1/6(pz)
  PS-Simulink Converter40/1 -> MATLAB Function1/7(vx)
  PS-Simulink Converter14/1 -> MATLAB Function2/5(py)
  PS-Simulink Converter46/1 -> MATLAB Function3/10(ax)
  MATLAB Function2/3(v) -> v1/1
  MATLAB Function1/3(v) -> v/1
  PS-Simulink Converter80/1 -> MATLAB Function1/11(ay)
  PS-Simulink Converter41/1 -> MATLAB Function1/8(vy)
  PS-Simulink Converter81/1 -> MATLAB Function1/12(az)
  PS-Simulink Converter48/1 -> MATLAB Function3/12(az)
  PS-Simulink Converter115/1 -> MATLAB Function2/11(ay)
  PS-Simulink Converter8/1 -> MATLAB Function1/5(py)
  MATLAB Function1/4(a) -> a/1
  MATLAB Function3/3(v) -> v2/1
  MATLAB Function3/2(p) -> p2/1
  MATLAB Function2/2(p) -> p1/1
  PS-Simulink Converter1/1 -> MATLAB Function1/1(bx)
  PS-Simulink Converter2/1 -> MATLAB Function1/2(by)
  PS-Simulink Converter3/1 -> MATLAB Function1/3(bz)
  PS-Simulink Converter4/1 -> MATLAB Function2/1(bx)
  PS-Simulink Converter5/1 -> MATLAB Function2/2(by)
  PS-Simulink Converter7/1 -> MATLAB Function2/3(bz)
  PS-Simulink Converter9/1 -> MATLAB Function3/1(bx)
  PS-Simulink Converter10/1 -> MATLAB Function3/2(by)
  PS-Simulink Converter11/1 -> MATLAB Function3/3(bz)
  MATLAB Function1/1(b) -> b/1
  MATLAB Function2/1(b) -> b1/1
  MATLAB Function3/1(b) -> b2/1
  connections:
  upperlegRF/RConn13 -- PS-Simulink Converter81/LConn1
  footRF/RConn9 -- PS-Simulink Converter17/LConn1
  upperlegRF/RConn10 -- PS-Simulink Converter42/LConn1
  lowerlegRF/RConn6 -- PS-Simulink Converter14/LConn1
  lowerlegRF/RConn9 -- PS-Simulink Converter44/LConn1
  footRF/LConn1 -- Conn1/RConn1
  lowerlegRF/RConn7 -- PS-Simulink Converter15/LConn1
  upperlegRF/RConn8 -- PS-Simulink Converter40/LConn1
  upperlegRF/RConn5 -- PS-Simulink Converter6/LConn1
  lowerlegRF/RConn5 -- PS-Simulink Converter13/LConn1
  lowerlegRF/RConn11 -- PS-Simulink Converter82/LConn1
  footRF/RConn12 -- PS-Simulink Converter47/LConn1
  lowerlegRF/RConn10 -- PS-Simulink Converter45/LConn1
  footRF/RConn13 -- PS-Simulink Converter48/LConn1
  lowerlegRF/RConn8 -- PS-Simulink Converter43/LConn1
  footRF/RConn10 -- PS-Simulink Converter18/LConn1
  upperlegRF/RConn9 -- PS-Simulink Converter41/LConn1
  upperlegRF/RConn11 -- PS-Simulink Converter79/LConn1
  footRF/RConn6 -- PS-Simulink Converter84/LConn1
  upperlegRF/RConn7 -- PS-Simulink Converter12/LConn1
  upperlegRF/LConn1 -- Conn2/RConn1
  footRF/RConn11 -- PS-Simulink Converter46/LConn1
  Conn5/RConn1 -- lowerlegRF/RConn1
  footRF/RConn1 -- Conn6/RConn1
  footRF/RConn7 -- PS-Simulink Converter85/LConn1
  footRF/RConn8 -- PS-Simulink Converter16/LConn1
  upperlegRF/RConn12 -- PS-Simulink Converter80/LConn1
  upperlegRF/RConn6 -- PS-Simulink Converter8/LConn1
  lowerlegRF/RConn13 -- PS-Simulink Converter116/LConn1
  lowerlegRF/LConn1 -- Conn3/RConn1
  footRF/RConn5 -- PS-Simulink Converter83/LConn1
  lowerlegRF/RConn12 -- PS-Simulink Converter115/LConn1
  upperlegRF/RConn1 -- Conn4/RConn1
  upperlegRF/RConn2 -- PS-Simulink Converter1/LConn1
  upperlegRF/RConn3 -- PS-Simulink Converter2/LConn1
  upperlegRF/RConn4 -- PS-Simulink Converter3/LConn1
  lowerlegRF/RConn2 -- PS-Simulink Converter4/LConn1
  lowerlegRF/RConn3 -- PS-Simulink Converter5/LConn1
  lowerlegRF/RConn4 -- PS-Simulink Converter7/LConn1
  footRF/RConn2 -- PS-Simulink Converter9/LConn1
  PS-Simulink Converter10/LConn1 -- footRF/RConn3
  footRF/RConn4 -- PS-Simulink Converter11/LConn1

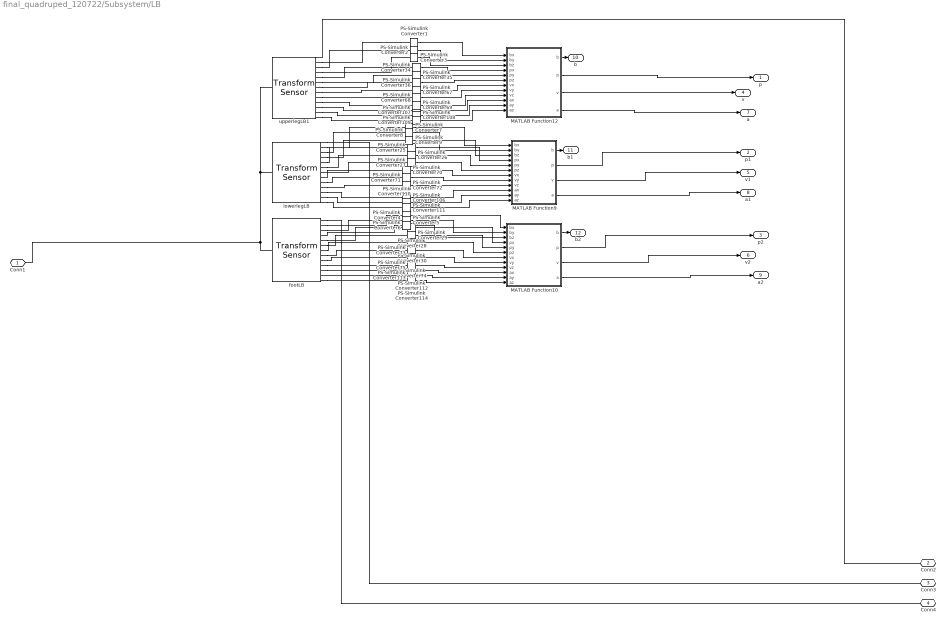
== system final_quadruped_120722/Subsystem/LB ==
  MATLAB Function10 : MATLAB Function  TreatAsAtomicUnit=on
  MATLAB Function12 : MATLAB Function  TreatAsAtomicUnit=on
  MATLAB Function9 : MATLAB Function  TreatAsAtomicUnit=on
  PS-Simulink Converter{1..9,25..30,34..36,67..75,106..114} (36 alike) : nesl_utility/PS-Simulink Converter  PhysicalDomain=network_engine_domain  SubClassName=ps_output  LeftPortType=input  RightPortType=output  PseudoPeriodic=off  Frequencies=[]  Unit=inherit  AffineConversion=off
      settings: SourceProductBaseCode=PW,SS
  footLB : sm_lib/Frames and Transforms/Transform Sensor  MeasurementFrame=World  SenseAngle=off  SenseAxis=off  SenseAngle1=off  SenseAngle2=off  SenseAngle3=off  SenseQ=off  SenseR=off  SenseOmegaX=off  SenseOmegaY=off  SenseOmegaZ=off  SenseOmega1=off  SenseOmega2=off  SenseOmega3=off  SenseQDot=off  SenseRDot=off  SenseAlphaX=on  SenseAlphaY=on  SenseAlphaZ=on  SenseAlpha1=off  SenseAlpha2=off  SenseAlpha3=off  SenseQDDot=off  SenseRDDot=off  SenseX=on  SenseY=on  SenseZ=on  SenseRad=off  SenseAzim=off  SenseDist=off  SenseInc=off  SenseXDot=on  SenseYDot=on  SenseZDot=on  SenseRadDot=off  SenseAzimDot=off  SenseDistDot=off  SenseIncDot=off  SenseXDDot=on  SenseYDDot=on  SenseZDDot=on  SenseRadDDot=off  SenseAzimDDot=off  SenseDistDDot=off  SenseIncDDot=off
  lowerlegLB : sm_lib/Frames and Transforms/Transform Sensor  MeasurementFrame=World  SenseAngle=off  SenseAxis=off  SenseAngle1=off  SenseAngle2=off  SenseAngle3=off  SenseQ=off  SenseR=off  SenseOmegaX=off  SenseOmegaY=off  SenseOmegaZ=off  SenseOmega1=off  SenseOmega2=off  SenseOmega3=off  SenseQDot=off  SenseRDot=off  SenseAlphaX=on  SenseAlphaY=on  SenseAlphaZ=on  SenseAlpha1=off  SenseAlpha2=off  SenseAlpha3=off  SenseQDDot=off  SenseRDDot=off  SenseX=on  SenseY=on  SenseZ=on  SenseRad=off  SenseAzim=off  SenseDist=off  SenseInc=off  SenseXDot=on  SenseYDot=on  SenseZDot=on  SenseRadDot=off  SenseAzimDot=off  SenseDistDot=off  SenseIncDot=off  SenseXDDot=on  SenseYDDot=on  SenseZDDot=on  SenseRadDDot=off  SenseAzimDDot=off  SenseDistDDot=off  SenseIncDDot=off
  upperlegLB1 : sm_lib/Frames and Transforms/Transform Sensor  MeasurementFrame=World  SenseAngle=off  SenseAxis=off  SenseAngle1=off  SenseAngle2=off  SenseAngle3=off  SenseQ=off  SenseR=off  SenseOmegaX=off  SenseOmegaY=off  SenseOmegaZ=off  SenseOmega1=off  SenseOmega2=off  SenseOmega3=off  SenseQDot=off  SenseRDot=off  SenseAlphaX=on  SenseAlphaY=on  SenseAlphaZ=on  SenseAlpha1=off  SenseAlpha2=off  SenseAlpha3=off  SenseQDDot=off  SenseRDDot=off  SenseX=on  SenseY=on  SenseZ=on  SenseRad=off  SenseAzim=off  SenseDist=off  SenseInc=off  SenseXDot=on  SenseYDot=on  SenseZDot=on  SenseRadDot=off  SenseAzimDot=off  SenseDistDot=off  SenseIncDot=off  SenseXDDot=on  SenseYDDot=on  SenseZDDot=on  SenseRadDDot=off  SenseAzimDDot=off  SenseDistDDot=off  SenseIncDDot=off
  Conn1 : PMIOPort  Side=Left
  Conn2 : PMIOPort  Port=2  Side=Right
  Conn3 : PMIOPort  Port=3  Side=Right
  Conn4 : PMIOPort  Port=4  Side=Right
  p : Outport
  p1 : Outport  Port=2
  p2 : Outport  Port=3
  v : Outport  Port=4
  v1 : Outport  Port=5
  v2 : Outport  Port=6
  a : Outport  Port=7
  a1 : Outport  Port=8
  a2 : Outport  Port=9
  b : Outport  Port=10
  b1 : Outport  Port=11
  b2 : Outport  Port=12
  wires:
  PS-Simulink Converter28/1 -> MATLAB Function10/4(px)
  PS-Simulink Converter108/1 -> MATLAB Function12/11(ay)
  PS-Simulink Converter36/1 -> MATLAB Function12/6(pz)
  PS-Simulink Converter114/1 -> MATLAB Function10/12(az)
  PS-Simulink Converter29/1 -> MATLAB Function10/5(py)
  PS-Simulink Converter75/1 -> MATLAB Function10/9(vz)
  PS-Simulink Converter109/1 -> MATLAB Function12/12(az)
  PS-Simulink Converter112/1 -> MATLAB Function10/10(ax)
  PS-Simulink Converter106/1 -> MATLAB Function9/10(ax)
  PS-Simulink Converter26/1 -> MATLAB Function9/5(py)
  PS-Simulink Converter67/1 -> MATLAB Function12/7(vx)
  PS-Simulink Converter35/1 -> MATLAB Function12/5(py)
  PS-Simulink Converter74/1 -> MATLAB Function10/8(vy)
  PS-Simulink Converter25/1 -> MATLAB Function9/4(px)
  MATLAB Function9/4(a) -> a1/1
  PS-Simulink Converter68/1 -> MATLAB Function12/8(vy)
  PS-Simulink Converter69/1 -> MATLAB Function12/9(vz)
  PS-Simulink Converter70/1 -> MATLAB Function9/7(vx)
  PS-Simulink Converter71/1 -> MATLAB Function9/8(vy)
  PS-Simulink Converter72/1 -> MATLAB Function9/9(vz)
  PS-Simulink Converter73/1 -> MATLAB Function10/7(vx)
  PS-Simulink Converter27/1 -> MATLAB Function9/6(pz)
  PS-Simulink Converter111/1 -> MATLAB Function9/12(az)
  PS-Simulink Converter30/1 -> MATLAB Function10/6(pz)
  MATLAB Function9/3(v) -> v1/1
  PS-Simulink Converter113/1 -> MATLAB Function10/11(ay)
  MATLAB Function10/3(v) -> v2/1
  PS-Simulink Converter110/1 -> MATLAB Function9/11(ay)
  PS-Simulink Converter34/1 -> MATLAB Function12/4(px)
  PS-Simulink Converter107/1 -> MATLAB Function12/10(ax)
  MATLAB Function12/3(v) -> v/1
  MATLAB Function10/4(a) -> a2/1
  MATLAB Function12/4(a) -> a/1
  MATLAB Function12/2(p) -> p/1
  MATLAB Function9/2(p) -> p1/1
  MATLAB Function10/2(p) -> p2/1
  PS-Simulink Converter1/1 -> MATLAB Function12/1(bx)
  PS-Simulink Converter2/1 -> MATLAB Function12/2(by)
  PS-Simulink Converter3/1 -> MATLAB Function12/3(bz)
  PS-Simulink Converter7/1 -> MATLAB Function9/1(bx)
  PS-Simulink Converter8/1 -> MATLAB Function9/2(by)
  PS-Simulink Converter9/1 -> MATLAB Function9/3(bz)
  PS-Simulink Converter4/1 -> MATLAB Function10/1(bx)
  PS-Simulink Converter5/1 -> MATLAB Function10/2(by)
  PS-Simulink Converter6/1 -> MATLAB Function10/3(bz)
  MATLAB Function12/1(b) -> b/1
  MATLAB Function9/1(b) -> b1/1
  MATLAB Function10/1(b) -> b2/1
  connections:
  PS-Simulink Converter113/LConn1 -- footLB/RConn12
  upperlegLB1/RConn6 -- PS-Simulink Converter35/LConn1
  lowerlegLB/RConn9 -- PS-Simulink Converter71/LConn1
  lowerlegLB/LConn1 -- upperlegLB1/LConn1 -- Conn1/RConn1 -- footLB/LConn1
  footLB/RConn7 -- PS-Simulink Converter30/LConn1
  lowerlegLB/RConn6 -- PS-Simulink Converter26/LConn1
  lowerlegLB/RConn8 -- PS-Simulink Converter70/LConn1
  footLB/RConn9 -- PS-Simulink Converter74/LConn1
  upperlegLB1/RConn13 -- PS-Simulink Converter109/LConn1
  upperlegLB1/RConn12 -- PS-Simulink Converter108/LConn1
  lowerlegLB/RConn13 -- PS-Simulink Converter111/LConn1
  lowerlegLB/RConn7 -- PS-Simulink Converter27/LConn1
  upperlegLB1/RConn8 -- PS-Simulink Converter67/LConn1
  upperlegLB1/RConn11 -- PS-Simulink Converter107/LConn1
  upperlegLB1/RConn5 -- PS-Simulink Converter34/LConn1
  footLB/RConn6 -- PS-Simulink Converter29/LConn1
  lowerlegLB/RConn12 -- PS-Simulink Converter110/LConn1
  lowerlegLB/RConn11 -- PS-Simulink Converter106/LConn1
  footLB/RConn5 -- PS-Simulink Converter28/LConn1
  upperlegLB1/RConn1 -- Conn2/RConn1
  footLB/RConn11 -- PS-Simulink Converter112/LConn1
  lowerlegLB/RConn10 -- PS-Simulink Converter72/LConn1
  upperlegLB1/RConn10 -- PS-Simulink Converter69/LConn1
  lowerlegLB/RConn5 -- PS-Simulink Converter25/LConn1
  footLB/RConn8 -- PS-Simulink Converter73/LConn1
  footLB/RConn10 -- PS-Simulink Converter75/LConn1
  upperlegLB1/RConn9 -- PS-Simulink Converter68/LConn1
  upperlegLB1/RConn7 -- PS-Simulink Converter36/LConn1
  footLB/RConn13 -- PS-Simulink Converter114/LConn1
  footLB/RConn1 -- Conn4/RConn1
  lowerlegLB/RConn1 -- Conn3/RConn1
  upperlegLB1/RConn2 -- PS-Simulink Converter1/LConn1
  upperlegLB1/RConn3 -- PS-Simulink Converter2/LConn1
  upperlegLB1/RConn4 -- PS-Simulink Converter3/LConn1
  lowerlegLB/RConn2 -- PS-Simulink Converter7/LConn1
  lowerlegLB/RConn3 -- PS-Simulink Converter8/LConn1
  lowerlegLB/RConn4 -- PS-Simulink Converter9/LConn1
  footLB/RConn2 -- PS-Simulink Converter4/LConn1
  footLB/RConn3 -- PS-Simulink Converter5/LConn1
  footLB/RConn4 -- PS-Simulink Converter6/LConn1

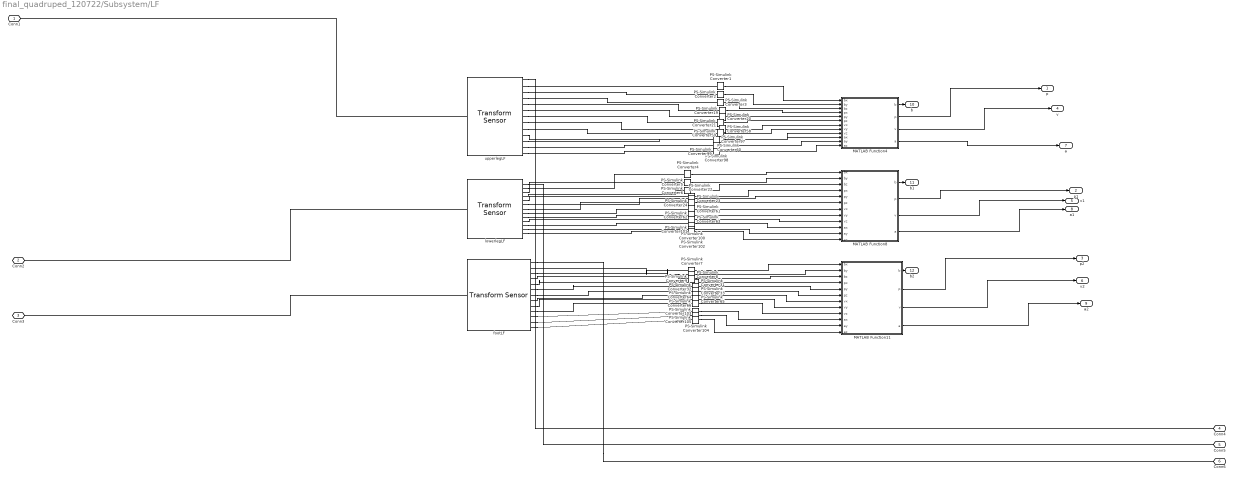
== system final_quadruped_120722/Subsystem/LF ==
  MATLAB Function11 : MATLAB Function  TreatAsAtomicUnit=on
  MATLAB Function4 : MATLAB Function  TreatAsAtomicUnit=on
  MATLAB Function8 : MATLAB Function  TreatAsAtomicUnit=on
  PS-Simulink Converter{1..9,19..24,31..33,58..66,97..105} (36 alike) : nesl_utility/PS-Simulink Converter  PhysicalDomain=network_engine_domain  SubClassName=ps_output  LeftPortType=input  RightPortType=output  PseudoPeriodic=off  Frequencies=[]  Unit=inherit  AffineConversion=off
      settings: SourceProductBaseCode=PW,SS
  footLF : sm_lib/Frames and Transforms/Transform Sensor  MeasurementFrame=World  SenseAngle=off  SenseAxis=off  SenseAngle1=off  SenseAngle2=off  SenseAngle3=off  SenseQ=off  SenseR=off  SenseOmegaX=off  SenseOmegaY=off  SenseOmegaZ=off  SenseOmega1=off  SenseOmega2=off  SenseOmega3=off  SenseQDot=off  SenseRDot=off  SenseAlphaX=on  SenseAlphaY=on  SenseAlphaZ=on  SenseAlpha1=off  SenseAlpha2=off  SenseAlpha3=off  SenseQDDot=off  SenseRDDot=off  SenseX=on  SenseY=on  SenseZ=on  SenseRad=off  SenseAzim=off  SenseDist=off  SenseInc=off  SenseXDot=on  SenseYDot=on  SenseZDot=on  SenseRadDot=off  SenseAzimDot=off  SenseDistDot=off  SenseIncDot=off  SenseXDDot=on  SenseYDDot=on  SenseZDDot=on  SenseRadDDot=off  SenseAzimDDot=off  SenseDistDDot=off  SenseIncDDot=off
  lowerlegLF : sm_lib/Frames and Transforms/Transform Sensor  MeasurementFrame=World  SenseAngle=off  SenseAxis=off  SenseAngle1=off  SenseAngle2=off  SenseAngle3=off  SenseQ=off  SenseR=off  SenseOmegaX=off  SenseOmegaY=off  SenseOmegaZ=off  SenseOmega1=off  SenseOmega2=off  SenseOmega3=off  SenseQDot=off  SenseRDot=off  SenseAlphaX=on  SenseAlphaY=on  SenseAlphaZ=on  SenseAlpha1=off  SenseAlpha2=off  SenseAlpha3=off  SenseQDDot=off  SenseRDDot=off  SenseX=on  SenseY=on  SenseZ=on  SenseRad=off  SenseAzim=off  SenseDist=off  SenseInc=off  SenseXDot=on  SenseYDot=on  SenseZDot=on  SenseRadDot=off  SenseAzimDot=off  SenseDistDot=off  SenseIncDot=off  SenseXDDot=on  SenseYDDot=on  SenseZDDot=on  SenseRadDDot=off  SenseAzimDDot=off  SenseDistDDot=off  SenseIncDDot=off
  upperlegLF : sm_lib/Frames and Transforms/Transform Sensor  MeasurementFrame=World  SenseAngle=off  SenseAxis=off  SenseAngle1=off  SenseAngle2=off  SenseAngle3=off  SenseQ=off  SenseR=off  SenseOmegaX=off  SenseOmegaY=off  SenseOmegaZ=off  SenseOmega1=off  SenseOmega2=off  SenseOmega3=off  SenseQDot=off  SenseRDot=off  SenseAlphaX=on  SenseAlphaY=on  SenseAlphaZ=on  SenseAlpha1=off  SenseAlpha2=off  SenseAlpha3=off  SenseQDDot=off  SenseRDDot=off  SenseX=on  SenseY=on  SenseZ=on  SenseRad=off  SenseAzim=off  SenseDist=off  SenseInc=off  SenseXDot=on  SenseYDot=on  SenseZDot=on  SenseRadDot=off  SenseAzimDot=off  SenseDistDot=off  SenseIncDot=off  SenseXDDot=on  SenseYDDot=on  SenseZDDot=on  SenseRadDDot=off  SenseAzimDDot=off  SenseDistDDot=off  SenseIncDDot=off
  Conn1 : PMIOPort  Side=Left
  Conn2 : PMIOPort  Port=2  Side=Left
  Conn3 : PMIOPort  Port=3  Side=Left
  Conn4 : PMIOPort  Port=4  Side=Right
  Conn5 : PMIOPort  Port=5  Side=Right
  Conn6 : PMIOPort  Port=6  Side=Right
  p : Outport
  p1 : Outport  Port=2
  p2 : Outport  Port=3
  v : Outport  Port=4
  v1 : Outport  Port=5
  v2 : Outport  Port=6
  a : Outport  Port=7
  a1 : Outport  Port=8
  a2 : Outport  Port=9
  b : Outport  Port=10
  b1 : Outport  Port=11
  b2 : Outport  Port=12
  wires:
  PS-Simulink Converter23/1 -> MATLAB Function8/5(py)
  MATLAB Function4/3(v) -> v/1
  PS-Simulink Converter100/1 -> MATLAB Function8/10(ax)
  PS-Simulink Converter20/1 -> MATLAB Function4/5(py)
  PS-Simulink Converter104/1 -> MATLAB Function11/11(ay)
  PS-Simulink Converter24/1 -> MATLAB Function8/6(pz)
  PS-Simulink Converter61/1 -> MATLAB Function8/7(vx)
  PS-Simulink Converter66/1 -> MATLAB Function11/9(vz)
  PS-Simulink Converter103/1 -> MATLAB Function11/10(ax)
  PS-Simulink Converter58/1 -> MATLAB Function4/7(vx)
  MATLAB Function4/4(a) -> a/1
  PS-Simulink Converter62/1 -> MATLAB Function8/8(vy)
  PS-Simulink Converter59/1 -> MATLAB Function4/8(vy)
  PS-Simulink Converter99/1 -> MATLAB Function4/12(az)
  MATLAB Function8/3(v) -> v1/1
  PS-Simulink Converter33/1 -> MATLAB Function11/6(pz)
  PS-Simulink Converter63/1 -> MATLAB Function8/9(vz)
  PS-Simulink Converter31/1 -> MATLAB Function11/4(px)
  PS-Simulink Converter22/1 -> MATLAB Function8/4(px)
  MATLAB Function8/4(a) -> a1/1
  PS-Simulink Converter102/1 -> MATLAB Function8/12(az)
  PS-Simulink Converter19/1 -> MATLAB Function4/4(px)
  PS-Simulink Converter97/1 -> MATLAB Function4/10(ax)
  PS-Simulink Converter101/1 -> MATLAB Function8/11(ay)
  PS-Simulink Converter64/1 -> MATLAB Function11/7(vx)
  PS-Simulink Converter65/1 -> MATLAB Function11/8(vy)
  MATLAB Function8/2(p) -> p1/1
  PS-Simulink Converter32/1 -> MATLAB Function11/5(py)
  PS-Simulink Converter105/1 -> MATLAB Function11/12(az)
  PS-Simulink Converter98/1 -> MATLAB Function4/11(ay)
  PS-Simulink Converter21/1 -> MATLAB Function4/6(pz)
  MATLAB Function11/4(a) -> a2/1
  PS-Simulink Converter60/1 -> MATLAB Function4/9(vz)
  MATLAB Function4/2(p) -> p/1
  MATLAB Function11/2(p) -> p2/1
  MATLAB Function11/3(v) -> v2/1
  PS-Simulink Converter1/1 -> MATLAB Function4/1(bx)
  PS-Simulink Converter2/1 -> MATLAB Function4/2(by)
  PS-Simulink Converter3/1 -> MATLAB Function4/3(bz)
  PS-Simulink Converter4/1 -> MATLAB Function8/1(bx)
  PS-Simulink Converter5/1 -> MATLAB Function8/2(by)
  PS-Simulink Converter6/1 -> MATLAB Function8/3(bz)
  PS-Simulink Converter7/1 -> MATLAB Function11/1(bx)
  PS-Simulink Converter8/1 -> MATLAB Function11/2(by)
  PS-Simulink Converter9/1 -> MATLAB Function11/3(bz)
  MATLAB Function4/1(b) -> b/1
  MATLAB Function8/1(b) -> b1/1
  MATLAB Function11/1(b) -> b2/1
  connections:
  footLF/RConn5 -- PS-Simulink Converter31/LConn1
  lowerlegLF/RConn10 -- PS-Simulink Converter63/LConn1
  upperlegLF/RConn5 -- PS-Simulink Converter19/LConn1
  upperlegLF/RConn12 -- PS-Simulink Converter98/LConn1
  upperlegLF/RConn8 -- PS-Simulink Converter58/LConn1
  upperlegLF/RConn11 -- PS-Simulink Converter97/LConn1
  footLF/RConn10 -- PS-Simulink Converter66/LConn1
  footLF/RConn6 -- PS-Simulink Converter32/LConn1
  lowerlegLF/RConn9 -- PS-Simulink Converter62/LConn1
  footLF/RConn7 -- PS-Simulink Converter33/LConn1
  lowerlegLF/RConn6 -- PS-Simulink Converter23/LConn1
  lowerlegLF/RConn13 -- PS-Simulink Converter102/LConn1
  footLF/RConn9 -- PS-Simulink Converter65/LConn1
  lowerlegLF/RConn7 -- PS-Simulink Converter24/LConn1
  footLF/RConn12 -- PS-Simulink Converter104/LConn1
  upperlegLF/RConn7 -- PS-Simulink Converter21/LConn1
  upperlegLF/RConn9 -- PS-Simulink Converter59/LConn1
  upperlegLF/LConn1 -- Conn1/RConn1
  lowerlegLF/RConn5 -- PS-Simulink Converter22/LConn1
  footLF/RConn8 -- PS-Simulink Converter64/LConn1
  upperlegLF/RConn10 -- PS-Simulink Converter60/LConn1
  footLF/RConn1 -- Conn6/RConn1
  upperlegLF/RConn6 -- PS-Simulink Converter20/LConn1
  footLF/RConn13 -- PS-Simulink Converter105/LConn1
  lowerlegLF/RConn11 -- PS-Simulink Converter100/LConn1
  lowerlegLF/RConn12 -- PS-Simulink Converter101/LConn1
  footLF/RConn11 -- PS-Simulink Converter103/LConn1
  lowerlegLF/RConn8 -- PS-Simulink Converter61/LConn1
  footLF/LConn1 -- Conn3/RConn1
  upperlegLF/RConn13 -- PS-Simulink Converter99/LConn1
  lowerlegLF/LConn1 -- Conn2/RConn1
  upperlegLF/RConn1 -- Conn4/RConn1
  lowerlegLF/RConn1 -- Conn5/RConn1
  upperlegLF/RConn2 -- PS-Simulink Converter1/LConn1
  upperlegLF/RConn3 -- PS-Simulink Converter2/LConn1
  upperlegLF/RConn4 -- PS-Simulink Converter3/LConn1
  lowerlegLF/RConn2 -- PS-Simulink Converter4/LConn1
  lowerlegLF/RConn3 -- PS-Simulink Converter5/LConn1
  lowerlegLF/RConn4 -- PS-Simulink Converter6/LConn1
  PS-Simulink Converter7/LConn1 -- footLF/RConn2
  footLF/RConn3 -- PS-Simulink Converter8/LConn1
  footLF/RConn4 -- PS-Simulink Converter9/LConn1
